simulink model "MCC"  (R2018b)
settings: Solver=VariableStepAuto  StartTime=0.0  StopTime=10  RelTol=1e-3
model workspace (MAT data in the model file):
  K = 0.45
undefined symbols (not defined in the file): f, J, L, R
settings Model: Creator=hp  LastModifiedBy=hp

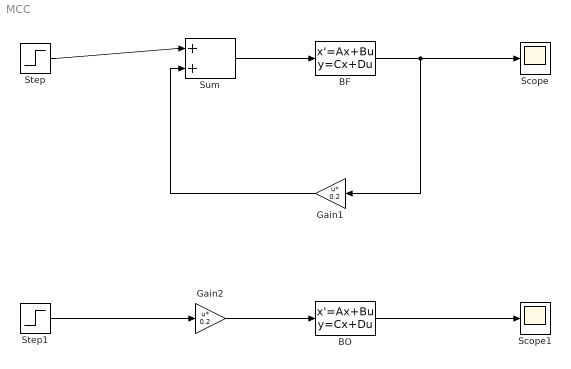
== system MCC ==
  BF : StateSpace  A=[-R/L 0; K/J -f/J]  B=[1/L ;0]  C=[1 0]  D=0  InitialCondition=0
  BO : StateSpace  A=[-R/L 0; K/J -f/J]  B=[1/L ;0]  C=[1 0]  D=0  InitialCondition=0
  Gain1 : Gain  Gain=0.2  Multiplication=Matrix(u*K)
  Gain2 : Gain  Gain=0.2  Multiplication=Matrix(u*K)
  Scope : Scope
  Scope1 : Scope
  Step : Step  SampleTime=0
  Step1 : Step  SampleTime=0
  Sum : Sum  Inputs=|++
  wires:
  Sum/1 -> BF/1
  BF/1 -> Gain1/1, Scope/1
  Gain1/1 -> Sum/2
  Gain2/1 -> BO/1
  BO/1 -> Scope1/1
  Step1/1 -> Gain2/1
  Step/1 -> Sum/1
